simulink model "LabProjectSimulink"  (R2017a)
settings: Solver=VariableStepAuto  StartTime=0.0  StopTime=inf  RelTol=1e-3
undefined symbols (not defined in the file or in its folder): fmRxParams, startfcn_spectrum_analyzer
libraries: simulink x2, dspsnks4 x1, commanabbnd3 x1, rtlsdr_book_library x1, dspmlti4 x1, sdrrlib x1
settings Model: Creator=Abdullah  LastModifiedBy=Abdullah

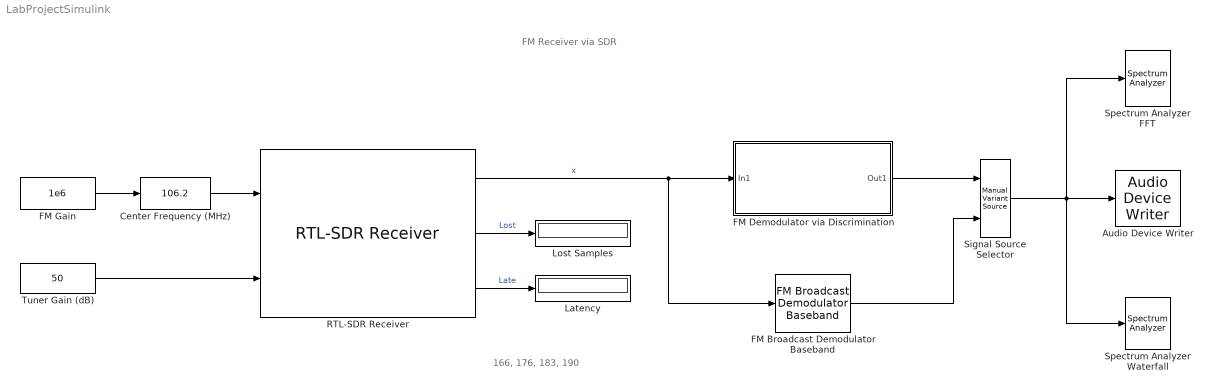
== system LabProjectSimulink ==
  note: FM Receiver via SDR
  note: 166, 176, 183, 190
  Audio Device Writer : dspsnks4/Audio Device Writer  Driver=DirectSound  Device=Default  InheritSampleRate=on  SampleRate=44100  BitDepth=16-bit integer  BufferSize=4096  NumBuffers=10  DefaultOutputChannelMapping=on  OutputChannelMapping=1:2  OutputNumUnderrunSamples=off  DriverIdx=1  DeviceWarnFlag=''
  Center Frequency (MHz) : simulink/Math Operations/Slider Gain  gain=106.2  low=87.9  high=107.9
  FM Broadcast Demodulator Baseband : commanabbnd3/FM Broadcast Demodulator Baseband  SampleRate=240e3  FrequencyDeviation=75e3  FilterTimeConstant=7.5e-5  AudioSampleRate=48e3  PlaySound=off  BufferSize=fmRxParams.BufferSize  Stereo=off  RBDS=off  RBDSSamplesPerSymbol=10  RBDSCostasLoop=off  SimulateUsing=Code generation
      settings: SourceProductName=Communications System Toolbox  SourceProductBaseCode=CM
  "FM Demodulator via Discrimination " : Subsystem
  FM Gain : Constant  Value=1e6  VectorParams1D=off  SampleTime=-1  FramePeriod=-1
  Latency : Display
  Lost Samples : Display
  RTL-SDR Receiver : sdrrlib/RTL-SDR Receiver  SourceLibraryInfo="This block requires <a href=\"http://www.mathworks.com/hardware-support/rtl-sdr.html\">Communications System Toolbox Support Package for RTL-SDR Radio</a>"  sobjType=sdrr.internal.SDRRTLReceiverSL  IPAddress=0  dataUDPPort=-1  ctrlUDPPort=-1  subDeviceList=nosubdev  sdrBlockType=SDRBlockTypeSLT.SDRRxBlock  requester=UNUSED_BY_SFCN  sdrExecutionMode=SDRExecutionModeSLT.ExecModeHW  LostSamplesOutputPort=on  OutputDataType=single  FrameLength=3.2e3  EnableBurstMode=off  NumFramesInBurst=20  BypassUserLogic=off  DecimatorSelect=DDC decimator  SourceSelect=RF data  SineAmplitude=16000  EnableInternalClock=off  BypassIQBalance=off  CenterFrequency=102.5e6  IFBandwidth=40e6  ADCRateSource=Dialog  ADCRate=240e3  CenterFrequencySource=Input port  GainSource=Input port  IntermediateFrequency=0  Gain=0  DecimationFactorSource=Dialog  DecimationFactor=512  RFFrequencyIsTunable=logical(1)  SampleTime=(3.2e3)/(240e3)  IFBandwidthSource=Dialog  SineFrequency=30000  BypassDCBlockingFilter=off  IntermediateFrequencySource=Dialog  IQBalanceCoefficients=64  SkipAllHardwareResetAndInitialization=off  EnableIQCalibrationTable=on  CacheIQCalibrationTable=off  EnableOffsetTuning=off  EnableRTLAGC=off  EnableTestMode=off  EnableTunerAGC=off  FrequencyCorrectionSource=Dialog  FrequencyCorrection=0  NumMLBuffers=128  NumUSBBuffers=16  LatencyOutputPort=on  RTLCrystalFrequency=28800000  TunerCrystalFrequency=28800000
      settings: SourceProductName=Communications System Toolbox Support Package for RTL-SDR Radio  SourceProductBaseCode=RTLSDR
  Signal Source Selector : simulink/Signal Routing/Manual Variant Source  NumChoices=2  OverrideUsingVariant=V_1
      settings: SourceProductName=Simulink
  Spectrum Analyzer FFT : SpectrumAnalyzer  StartFcn=startfcn_spectrum_analyzer;
  Spectrum Analyzer Waterfall : SpectrumAnalyzer  StartFcn=startfcn_spectrum_analyzer;
  Tuner Gain (dB) : Constant  Value=50
  wires:
  Center Frequency (MHz)/1 -> RTL-SDR Receiver/1
  FM Gain/1 -> Center Frequency (MHz)/1
  RTL-SDR Receiver/3 -> Latency/1  "Late"
  RTL-SDR Receiver/2 -> Lost Samples/1  "Lost"
  Tuner Gain (dB)/1 -> RTL-SDR Receiver/2
  Signal Source Selector/1 -> Spectrum Analyzer Waterfall/1, Spectrum Analyzer FFT/1, Audio Device Writer/1
  RTL-SDR Receiver/1 -> FM Broadcast Demodulator Baseband/1, "FM Demodulator via Discrimination "/1(In1)  "x"
  FM Broadcast Demodulator Baseband/1 -> Signal Source Selector/2
  "FM Demodulator via Discrimination "/1(Out1) -> Signal Source Selector/1

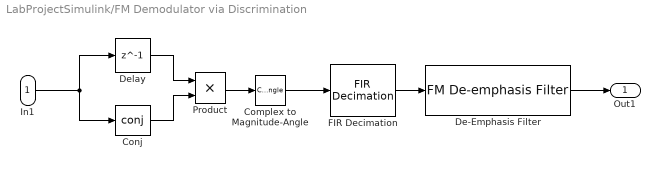
== system LabProjectSimulink/FM Demodulator via Discrimination  ==
  In1 : Inport
  Complex to Magnitude-Angle : ComplexToMagnitudeAngle  Output=Angle
  Conj : Math  Operator=conj  SaturateOnIntegerOverflow=on
  De-Emphasis Filter : rtlsdr_book_library/FM Demod Tools/FM De-emphasis Filter  region=Europe, Asia  fs=48e3
      settings: SourceProductName=RTL-SDR Book Library
  Delay : Delay  DelayLength=1  InitialCondition=0  InputProcessing=Columns as channels (frame based)
  "FIR Decimation " : dspmlti4/FIR Decimation  FilterSource=Dialog parameters  h=firpm(100, [0 15e3 20e3 (240e3/2)]/(240e3/2), [1 1 0 0], [1 1],20)  D=5  filtStruct=Direct form  FilterObject=Hm_firdecim  InputProcessing=Columns as channels (frame based)  framing=Allow multirate processing  inputOffset=0  outputBufInitCond=0  roundingMode=Floor  overflowMode=off  firstCoeffDataTypeStr=Inherit: Same word length as input  firstCoeffMin=[]  firstCoeffMax=[]  firstCoeffLastDataTypeStr=Inherit: Same word length as input  outputDataTypeStr=Inherit: Same as accumulator  outputMin=[]  outputMax=[]  outputLastDataTypeStr=Inherit: Same as accumulator
  Product : Product
  Out1 : Outport
  wires:
  De-Emphasis Filter/1 -> Out1/1
  In1/1 -> Conj/1, Delay/1
  Complex to Magnitude-Angle/1 -> "FIR Decimation "/1
  Product/1 -> Complex to Magnitude-Angle/1
  Conj/1 -> Product/2
  "FIR Decimation "/1 -> De-Emphasis Filter/1
  Delay/1 -> Product/1
